simulink model "EngineMap"  (R2018b)
settings: configuration reference "Physics" (kept outside this file)
model workspace (MAT data in the model file):
  veh_param = Simulink.Parameter
  veh_param.Value.cLiftF = 0
  veh_param.Value.cLiftR = 0
  veh_param.Value.CoGx_m = 0
  veh_param.Value.CoGy_m = 0
  veh_param.Value.CoGz_m = 0
  veh_param.Value.cDrag = 0
  veh_param.Value.Aref_m2 = 0
  veh_param.Value.Gearratio = 0
  veh_param.Value.Wheelbase_m = 0
  veh_param.Value.PacLatF = [0 0 0 0 0]
  veh_param.Value.PacLongF = [0 0 0 0 0]
  veh_param.Value.PacLatR = [0 0 0 0 0]
  veh_param.Value.PacLongR = [0 0 0 0 0]
  veh_param.Value.cRollFriction_Npmps = 0
  veh_param.Value.MaxRollFriction_N = 0
  veh_param.Value.T_YawRate_s = 0
  veh_param.Value.T_LatVel_s = 0
  veh_param.Value.TrackWidthF_m = 0
  veh_param.Value.TrackWidthR_m = 0
  veh_param.Value.TireRadiusF_m = 0
  veh_param.Value.TireRadiusR_m = 0
  veh_param.Value.VehicleInertia_kgm2 = 0
  veh_param.Value.WheelInertiaF_kgm2 = 0
  veh_param.Value.WheelInertiaR_kgm2 = 0
  veh_param.Value.VehicleMass_kg = 0
  veh_param.Value.switchModelBlend_mps = 0
  veh_param.Value.PTLimitLowVel_N = 0
  veh_param.Value.switchModelVel_mps = 0
  veh_param.Value.T_Tire_s = 0
  veh_param.DataType = 'struct'
  veh_param.Dimensions = [1 1]
  x0_positionstates = Simulink.Parameter
  x0_positionstates.Value = [0 0 0]
  x0_positionstates.DataType = 'auto'
  x0_positionstates.Dimensions = [1 3]
settings Model: DataDictionary=vehicleparameters_vehdynsim.sldd  OrderedModelArguments=off  Creator=wischnewski  LastModifiedBy=staer

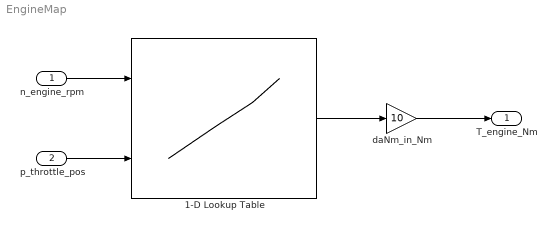
== system EngineMap ==
  n_engine_rpm : Inport
  p_throttle_pos : Inport  Port=2
  1-D Lookup Table : Lookup_n-D  BreakpointsForDimension1=[500,1500,2500,6300,6600,6900,7200,7500,7800,8100,8400,8700,9000,9300,9600,9900,10200]  BreakpointsForDimension2=[0,0.1,0.2,0.3,0.4,0.5,0.6,0.7,0.8,0.9,1]  Table=reshape([0,0,-5.7,-7.6,-9.5,-11.4,-13.3,-15.2,-17.1,-19,-22.8,-24.7,-24.7,-26.6,-27.55,-28.5,-30.4,1.9,1.9,0,0,1.9,3.8,1.9,3.8,1.9,0,-3.8,-5.7,-6.65,-7.6,-9.5,-10.45,-11.4,1.9,3.8,1.9,1.9,3.8,7.6,11.4,15.2,11.4,7.6,3.8,1.9,0,-1.9,-2.85,-3.8,-5.7,3.8,5.7,5.7,7.6,9.5,13.3,17.1,19,17.1,13.3,9.5,7.6,5.7,1.9,0,-1.9,-3.8,5.7,7.6,7.6,9.5,11.4,15.2,19,20.9,19,15.2,11.4,9.5,5.7,3.8,1.9,0,0,9.5,13.3,15.2,19,20.9,22.8,26.6,28.5,26.6,22.8,19,15.2,13.3,11.4,9.5,7.6,5.7,17.1,20.9,24.7,26.6,28.5,30.4,34.2,36.1,34.2,30.4,28.5,24.7,22.8,20.9,19,17.1,14.25,22.8,26.6,30.4,32.3,34.2,36.1,38,39.9,38,36.1,32.3,28.5,26.6,24.7,22.8,20.9,19,24.7,30.4,34.2,36.1,38,39.9,43.7,44.65,43.7,39.9,38,34.2,32.3,30.4,28.5,26.6,24.7,38,41.8,45.6,47.5,47.5,49.4,51.3,52.25,51.3,48.45,47.5,45.6,43.7,41.8,39.9,37.05,32.3,43.7,47.5,49.97,51.3,51.3,51.11,52.25,53.01,52.25,51.3,50.16,49.02,47.31,44.65,42.56,40.66,38],17,11)  InternalRulePriority=Speed  RndMeth=Simplest  InputSameDT=on
  daNm_in_Nm : Gain  Gain=10
  T_engine_Nm : Outport
  wires:
  n_engine_rpm/1 -> 1-D Lookup Table/1
  p_throttle_pos/1 -> 1-D Lookup Table/2
  1-D Lookup Table/1 -> daNm_in_Nm/1
  daNm_in_Nm/1 -> T_engine_Nm/1
